simulink model "accel_limit_test"  (R2025b)
settings: Solver=FixedStepDiscrete  StartTime=0.0  StopTime=10.0  FixedStep=1e-2  RelTol=1e-3
undefined symbols (not defined in the file or in its folder): DiscIntNeverNeededParam
libraries: simulink x3
settings Model: Creator=karadeli  LastModifiedBy=karadeli

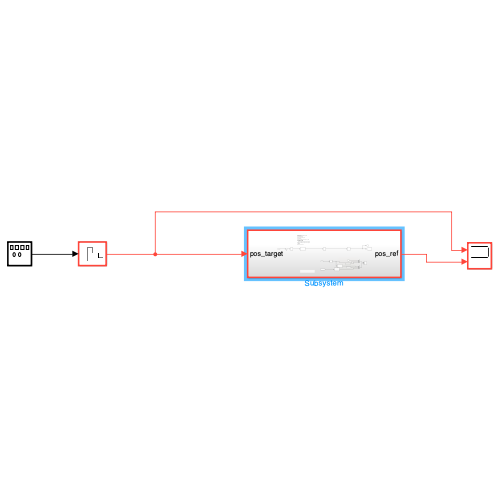
[thumbnail: Simulink's stored preview of the top-level diagram]
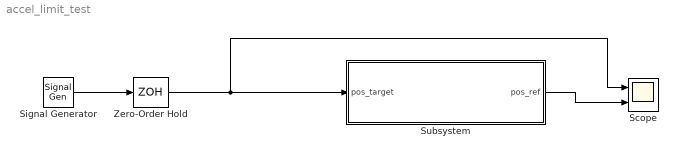
== system accel_limit_test ==
  Scope : Scope  NumInputPorts=2
      settings: ActiveDisplayYMinimum=-2497.7186917769627  ActiveDisplayYMaximum=2499.7465213085516
  Signal Generator : SignalGenerator  WaveForm=sawtooth  Amplitude=2000  Units=rad/sec
  Subsystem : Subsystem
  Zero-Order Hold : ZeroOrderHold  SampleTime=-1
  wires:
  Signal Generator/1 -> Zero-Order Hold/1
  Subsystem/1(pos_ref) -> Scope/2
  Zero-Order Hold/1 -> Scope/1, Subsystem/1(pos_target)

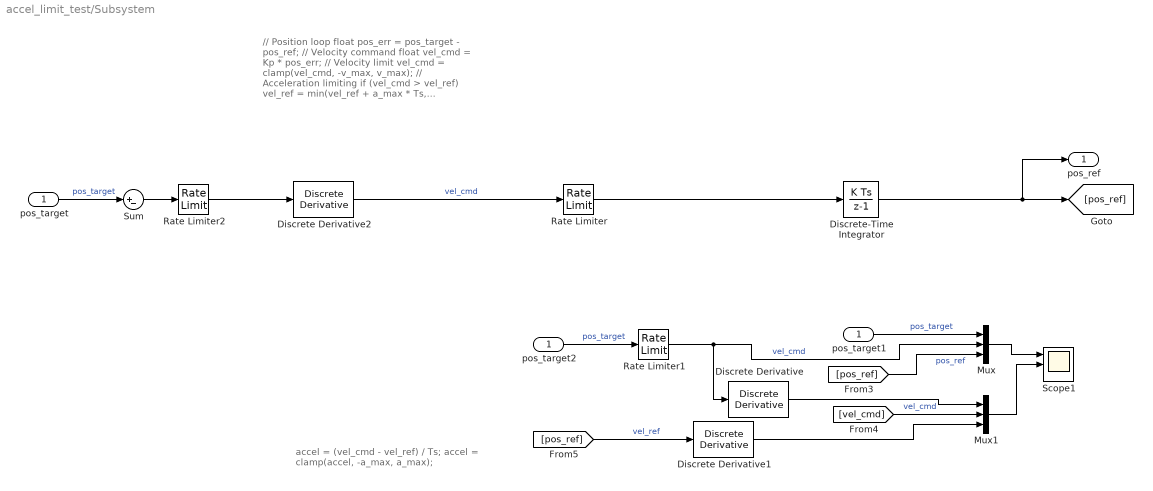
== system accel_limit_test/Subsystem ==
  note: accel = (vel_cmd - vel_ref) / Ts;
      | accel = clamp(accel, -a_max, a_max);
  note: // Position loop
      | float pos_err = pos_target - pos_ref;
      |
      | // Velocity command
      | float vel_cmd = Kp * pos_err;
      |
      | // Velocity limit
      | vel_cmd = clamp(vel_cmd, -v_max, v_max);
      |
      | // Acceleration limiting
      | if (vel_cmd > vel_ref)
      | vel_ref = min(vel_ref + a_max * Ts, vel_cmd);
      | else
      | vel_ref = max(vel_ref - a_max * Ts, vel_cmd);
      |
      | // Integrate
      | pos_ref += vel_ref * Ts;
  pos_target : Inport
  Discrete Derivative : simulink/Discrete/Discrete Derivative  gainval=1  ICPrevScaledInput=0.0  OutMin=[]  OutMax=[]  OutDataType=fixdt(1, 16)  OutScaling=2^-10  DoSatur=off
  Discrete Derivative1 : simulink/Discrete/Discrete Derivative  gainval=1  ICPrevScaledInput=0.0  OutMin=[]  OutMax=[]  OutDataType=fixdt(1, 16)  OutScaling=2^-10  DoSatur=off
  Discrete Derivative2 : simulink/Discrete/Discrete Derivative  gainval=1.0  ICPrevScaledInput=0.0  OutMin=[]  OutMax=[]  OutDataType=fixdt(1, 16)  OutScaling=2^-10  DoSatur=off
  Discrete-Time Integrator : DiscreteIntegrator  SampleTime=-1  ICPrevOutput=DiscIntNeverNeededParam  ICPrevScaledInput=DiscIntNeverNeededParam
  Mux : Mux  Inputs=3
  Mux1 : Mux  Inputs=3
  Rate Limiter : RateLimiter  RisingSlewLimit=1e4  FallingSlewLimit=-1e4  SampleTimeMode=inherited
  Rate Limiter1 : RateLimiter  RisingSlewLimit=2400  FallingSlewLimit=-2400  SampleTimeMode=inherited
  Rate Limiter2 : RateLimiter  RisingSlewLimit=2400  FallingSlewLimit=-2400  SampleTimeMode=inherited
  Scope1 : Scope  NumInputPorts=3
      settings: ActiveDisplayYMinimum=-2497.7186917769627  ActiveDisplayYMaximum=2499.7465213085516  DataLoggingVariableName=ScopeData2
  Sum : Sum  Inputs=|+-
  pos_target1 : InportShadow
  pos_target2 : InportShadow
  pos_ref : Outport
  wires:
  Discrete Derivative2/1 -> Rate Limiter/1  "vel_cmd"
  Rate Limiter/1 -> Discrete-Time Integrator/1
  pos_target/1 -> Sum/1  "pos_target"
  [pos_ref] -> Mux/3  "pos_ref"
  pos_target1/1 -> Mux/1  "pos_target"
  [vel_cmd] -> Mux1/2  "vel_cmd"
  [pos_ref] -> Discrete Derivative1/1  "vel_ref"
  Mux/1 -> Scope1/1
  Mux1/1 -> Scope1/2
  Discrete Derivative/1 -> Mux1/1
  Discrete Derivative1/1 -> Mux1/3
  pos_target2/1 -> Rate Limiter1/1  "pos_target"
  Rate Limiter1/1 -> Discrete Derivative/1, Mux/2  "vel_cmd"
  Rate Limiter2/1 -> Discrete Derivative2/1
  Discrete-Time Integrator/1 -> [pos_ref], pos_ref/1
  Sum/1 -> Rate Limiter2/1
